simulink model "course project"  (R2023b)
settings: Solver=VariableStepAuto  StartTime=0.0  StopTime=2  RelTol=1e-3
libraries: simulink x1
(part 1 of 2)
settings Model: Creator=1234  LastModifiedBy=1234

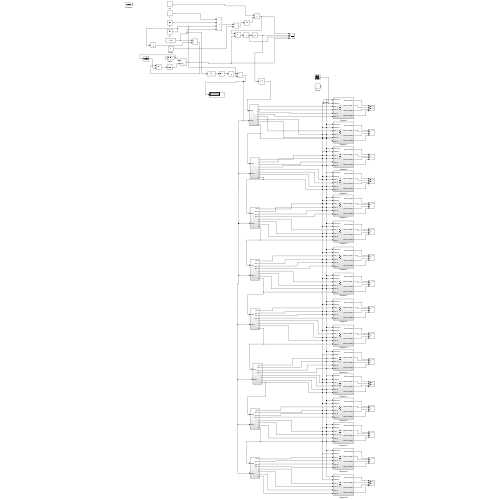
[thumbnail: Simulink's stored preview of the top-level diagram]
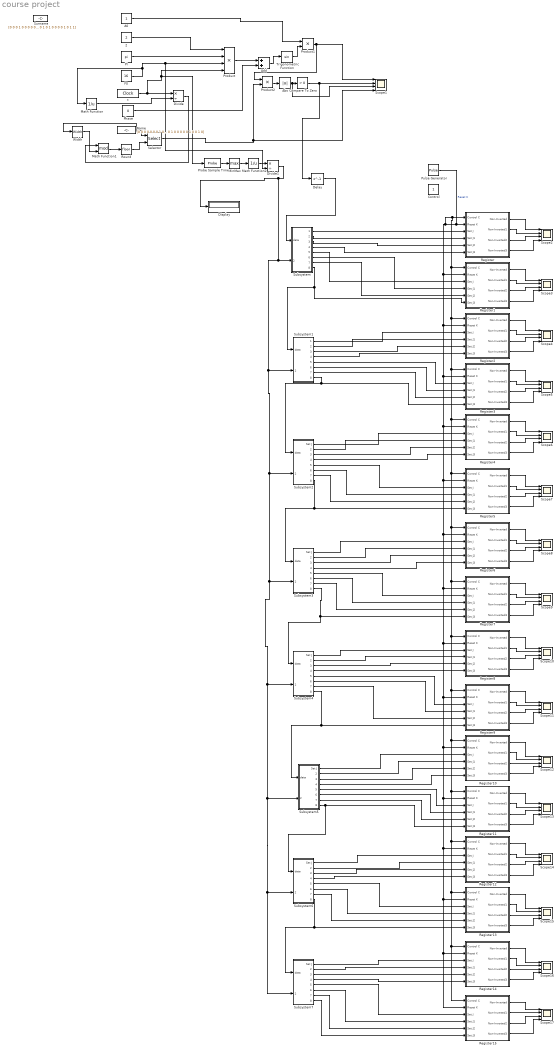
== system course project ==
  2 : Constant  Value=2
  A0 : Constant
  Abs : Abs  SaturateOnIntegerOverflow=off
  Add : Sum
  Compare To Zero : simulink/Logic and Bit Operations/Compare To Zero  relop=>  OutDataTypeStr=boolean
  Control : Constant
  Delay : Delay  DelayLength=1  InitialCondition=0
  Display : Display
  Divide : Product  Inputs=*/
  Divide1 : Product  Inputs=*/
  F0 : Constant  Value=16
  Math Function : Math  Operator=reciprocal
  Math Function1 : Math  Operator=mod
  Math Function2 : Math  Operator=reciprocal
  MinMax : MinMax  Function=max
  Name : Constant  Value=[0 0 0 0 0 0 0 1 0 0 0 0 1 1 0 0 0 0 0 0 0 1 0 1 0 0 0 1 1 0 0 0 0 0 0 0 0 0 0 1 0 0 0 0 1 1 1 0 0 0 0 0 0 1 0 0 0 0 0 1 0 0 1 0]  VectorParams1D=off
  PI : Constant  Value=pi
  Phase : Constant  Value=0
  Probe Sample Time : Probe  ProbeWidth=off  ProbeComplexSignal=off
  Product : Product  Inputs=4
  Product1 : Product
  Product2 : Product
  Pulse Generator : DiscretePulseGenerator  PulseType=Time based  PulseWidth=50
  Register : Subsystem
  Register1 : Subsystem
  Register10 : Subsystem
  Register11 : Subsystem
  Register12 : Subsystem
  Register13 : Subsystem
  Register14 : Subsystem
  Register15 : Subsystem
  Register2 : Subsystem
  Register3 : Subsystem
  Register4 : Subsystem
  Register5 : Subsystem
  Register6 : Subsystem
  Register7 : Subsystem
  Register8 : Subsystem
  Register9 : Subsystem
  Round : Rounding
  Scope{1..17} (17 alike) : Scope  NumInputPorts=4
  Selector : Selector  IndexMode=Zero-based  InputPortWidth=64  IndexOptions=Index vector (port)  Indices=[1 3]  OutputSizes=1
  Subsystem : Subsystem
  Subsystem1 : Subsystem
  Subsystem2 : Subsystem
  Subsystem3 : Subsystem
  Subsystem4 : Subsystem
  Subsystem5 : Subsystem
  Subsystem6 : Subsystem
  Subsystem7 : Subsystem
  Surname : Constant  Value=[0 0 0 1 0 0 0 0 0 0 0 0 1 1 1 1 0 0 0 0 0 1 1 1 0 0 0 1 0 0 1 0 0 0 0 0 0 1 0 1 0 0 0 0 0 0 1 0 0 0 0 0 1 1 1 0 0 0 0 1 1 0 0 1 0 0 0 1 0 1 0 1 0 0 0 0 1 0 1 1]
  Trigonometric Function : Trigonometry
  Width : Width
  t : DigitalClock  SampleTime=1/1000
  wires:
  Subsystem4/8(Out8) -> Register9/6(Set J3), Subsystem5/1(data)
  Trigonometric Function/1 -> Product1/2
  PI/1 -> Product/2
  A0/1 -> Product1/1
  MinMax/1 -> Math Function2/1
  Math Function1/1 -> Round/1
  Probe Sample Time/1 -> MinMax/1
  Product/1 -> Add/1
  Selector/1 -> Product2/2, Scope1/4
  Abs/1 -> Scope1/3, Compare To Zero/1
  Name/1 -> Width/1, Selector/1
  Subsystem1/8(Out8) -> Subsystem2/1(data), Register3/6(Set J3)
  Product2/1 -> Abs/1
  Product1/1 -> Scope1/1, Product2/1
  Phase/1 -> Add/2
  Subsystem6/8(Out8) -> Register13/6(Set J3), Subsystem7/1(data)
  Width/1 -> Math Function1/2
  Divide/1 -> Math Function1/1
  Math Function/1 -> Divide/2
  Compare To Zero/1 -> Delay/1, Scope1/2
  Round/1 -> Selector/2
  t/1 -> Probe Sample Time/1, Product/4, Divide/1
  2/1 -> Product/1
  Math Function2/1 -> Divide1/1
  F0/1 -> Math Function/1, Divide1/2, Product/3
  Subsystem/8(Out8) -> Register1/6(Set J3), Subsystem1/1(data)
  Delay/1 -> Subsystem/1(data)
  Subsystem5/8(Out8) -> Subsystem6/1(data), Register11/6(Set J3)
  Add/1 -> Trigonometric Function/1
  Subsystem2/8(Out8) -> Register5/6(Set J3), Subsystem3/1(data)
  Subsystem3/8(Out8) -> Register7/6(Set J3), Subsystem4/1(data)
  Subsystem/1(1) -> Register/3(Set J)
  Subsystem/2(2) -> Register/4(Set J1)
  Subsystem/3(3) -> Register/5(Set J2)
  Subsystem/4(4) -> Register/6(Set J3)
  Subsystem/5(Out5) -> Register1/3(Set J)
  Subsystem/6(Out6) -> Register1/4(Set J1)
  Subsystem/7(Out7) -> Register1/5(Set J2)
  Subsystem1/1(1) -> Register2/3(Set J)
  Subsystem1/2(2) -> Register2/4(Set J1)
  Subsystem1/3(3) -> Register2/5(Set J2)
  Subsystem1/4(4) -> Register2/6(Set J3)
  Subsystem1/5(Out5) -> Register3/3(Set J)
  Subsystem1/6(Out6) -> Register3/4(Set J1)
  Subsystem1/7(Out7) -> Register3/5(Set J2)
  Subsystem2/1(Set J) -> Register4/3(Set J)
  Subsystem2/2(Set J1) -> Register4/4(Set J1)
  Subsystem2/3(Set J2) -> Register4/5(Set J2)
  Subsystem2/4(Set J3) -> Register4/6(Set J3)
  Subsystem2/5(Out5) -> Register5/3(Set J)
  Subsystem2/6(Out6) -> Register5/4(Set J1)
  Subsystem2/7(Out7) -> Register5/5(Set J2)
  Subsystem3/1(Set J) -> Register6/3(Set J)
  Subsystem3/2(Set J1) -> Register6/4(Set J1)
  Subsystem3/3(Set J2) -> Register6/5(Set J2)
  Subsystem3/4(Set J3) -> Register6/6(Set J3)
  Subsystem3/5(Out5) -> Register7/3(Set J)
  Subsystem3/6(Out6) -> Register7/4(Set J1)
  Subsystem3/7(Out7) -> Register7/5(Set J2)
  Subsystem4/1(Set J) -> Register8/3(Set J)
  Subsystem4/2(Set J1) -> Register8/4(Set J1)
  Subsystem4/3(Set J2) -> Register8/5(Set J2)
  Subsystem4/4(Set J3) -> Register8/6(Set J3)
  Subsystem4/5(Out5) -> Register9/3(Set J)
  Subsystem4/6(Out6) -> Register9/4(Set J1)
  Subsystem4/7(Out7) -> Register9/5(Set J2)
  Subsystem5/1(Set J) -> Register10/3(Set J)
  Subsystem5/2(Set J1) -> Register10/4(Set J1)
  Subsystem5/3(Set J2) -> Register10/5(Set J2)
  Subsystem5/4(Set J3) -> Register10/6(Set J3)
  Subsystem5/5(Out5) -> Register11/3(Set J)
  Subsystem5/6(Out6) -> Register11/4(Set J1)
  Subsystem5/7(Out7) -> Register11/5(Set J2)
  Subsystem6/1(Set J) -> Register12/3(Set J)
  Subsystem6/2(Set J1) -> Register12/4(Set J1)
  Subsystem6/3(Set J2) -> Register12/5(Set J2)
  Subsystem6/4(Set J3) -> Register12/6(Set J3)
  Subsystem6/5(Out5) -> Register13/3(Set J)
  Subsystem6/6(Out6) -> Register13/4(Set J1)
  Subsystem6/7(Out7) -> Register13/5(Set J2)
  Subsystem7/1(Set J) -> Register14/3(Set J)
  Subsystem7/2(Set J1) -> Register14/4(Set J1)
  Subsystem7/3(Set J2) -> Register14/5(Set J2)
  Subsystem7/4(Set J3) -> Register14/6(Set J3)
  Subsystem7/5(Out5) -> Register15/3(Set J)
  Subsystem7/6(Out6) -> Register15/4(Set J1)
  Subsystem7/7(Out7) -> Register15/5(Set J2)
  Subsystem7/8(Out8) -> Register15/6(Set J3)
  Register/1(Non-Inverted) -> Scope2/1
  Register/2(Non-Inverted1) -> Scope2/2
  Register/3(Non-Inverted2) -> Scope2/3
  Register/4(Non-Inverted3) -> Scope2/4
  Register1/3(Non-Inverted2) -> Scope3/3
  Register1/4(Non-Inverted3) -> Scope3/4
  Register1/2(Non-Inverted1) -> Scope3/2
  Register1/1(Non-Inverted) -> Scope3/1
  Register2/3(Non-Inverted2) -> Scope4/3
  Register2/4(Non-Inverted3) -> Scope4/4
  Register2/2(Non-Inverted1) -> Scope4/2
  Register2/1(Non-Inverted) -> Scope4/1
  Register3/3(Non-Inverted2) -> Scope5/3
  Register3/4(Non-Inverted3) -> Scope5/4
  Register3/2(Non-Inverted1) -> Scope5/2
  Register3/1(Non-Inverted) -> Scope5/1
  Register4/3(Non-Inverted2) -> Scope6/3
  Register4/4(Non-Inverted3) -> Scope6/4
  Register4/2(Non-Inverted1) -> Scope6/2
  Register4/1(Non-Inverted) -> Scope6/1
  Register5/3(Non-Inverted2) -> Scope7/3
  Register5/4(Non-Inverted3) -> Scope7/4
  Register5/2(Non-Inverted1) -> Scope7/2
  Register5/1(Non-Inverted) -> Scope7/1
  Register6/3(Non-Inverted2) -> Scope8/3
  Register6/4(Non-Inverted3) -> Scope8/4
  Register6/2(Non-Inverted1) -> Scope8/2
  Register6/1(Non-Inverted) -> Scope8/1
  Register7/3(Non-Inverted2) -> Scope9/3
  Register7/4(Non-Inverted3) -> Scope9/4
  Register7/2(Non-Inverted1) -> Scope9/2
  Register7/1(Non-Inverted) -> Scope9/1
  Register8/3(Non-Inverted2) -> Scope10/3
  Register8/4(Non-Inverted3) -> Scope10/4
  Register8/2(Non-Inverted1) -> Scope10/2
  Register8/1(Non-Inverted) -> Scope10/1
  Register9/3(Non-Inverted2) -> Scope11/3
  Register9/4(Non-Inverted3) -> Scope11/4
  Register9/2(Non-Inverted1) -> Scope11/2
  Register9/1(Non-Inverted) -> Scope11/1
  Register10/1(Non-Inverted) -> Scope12/1
  Register10/2(Non-Inverted1) -> Scope12/2
  Register10/3(Non-Inverted2) -> Scope12/3
  Register10/4(Non-Inverted3) -> Scope12/4
  Register11/1(Non-Inverted) -> Scope13/1
  Register11/2(Non-Inverted1) -> Scope13/2
  Register11/3(Non-Inverted2) -> Scope13/3
  Register11/4(Non-Inverted3) -> Scope13/4
  Register15/1(Non-Inverted) -> Scope17/1
  Register15/2(Non-Inverted1) -> Scope17/2
  Register15/4(Non-Inverted3) -> Scope17/4
  Register14/4(Non-Inverted3) -> Scope16/4
  Register14/1(Non-Inverted) -> Scope16/1
  Register14/2(Non-Inverted1) -> Scope16/2
  Register14/3(Non-Inverted2) -> Scope16/3
  Register15/3(Non-Inverted2) -> Scope17/3
  Register12/2(Non-Inverted1) -> Scope14/2
  Register12/1(Non-Inverted) -> Scope14/1
  Register13/1(Non-Inverted) -> Scope15/1
  Register13/2(Non-Inverted1) -> Scope15/2
  Register12/4(Non-Inverted3) -> Scope14/4
  Register13/3(Non-Inverted2) -> Scope15/3
  Register12/3(Non-Inverted2) -> Scope14/3
  Register13/4(Non-Inverted3) -> Scope15/4
  Divide1/1 -> Display/1, Subsystem7/2(delay), Subsystem6/2(delay), Subsystem5/2(delay), Subsystem4/2(delay), Subsystem3/2(delay), Subsystem2/2(delay), Subsystem1/2(delay), Subsystem/2(delay)
  Pulse Generator/1 -> Register1/1(Control C), Register2/1(Control C), Register3/1(Control C), Register4/1(Control C), Register5/1(Control C), Register6/1(Control C), Register7/1(Control C), Register8/1(Control C), Register9/1(Control C), Register10/1(Control C), Register11/1(Control C), Register12/1(Control C), Register13/1(Control C), Register14/1(Control C), Register15/1(Control C), Register/1(Control C), Register15/2(Reset K), Register14/2(Reset K), Register13/2(Reset K), Register12/2(Reset K), Register11/2(Reset K), Register10/2(Reset K), Register9/2(Reset K), Register8/2(Reset K), Register7/2(Reset K), Register6/2(Reset K), Register5/2(Reset K), Register4/2(Reset K), Register3/2(Reset K), Register2/2(Reset K), Register1/2(Reset K), Register/2(Reset K)  "Reset K"

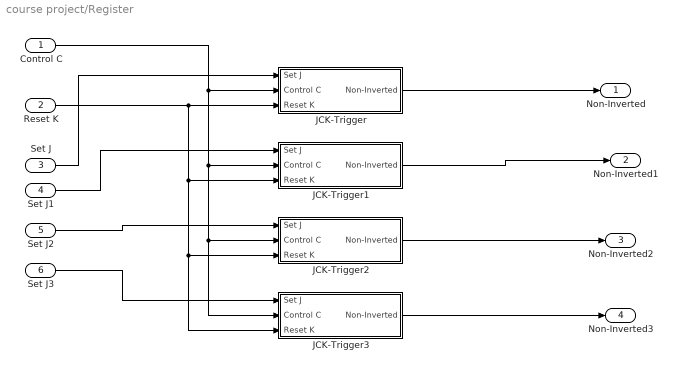
== system course project/Register ==
  Control C : Inport
  Reset K : Inport  Port=2
  Set J : Inport  Port=3
  Set J1 : Inport  Port=4
  Set J2 : Inport  Port=5
  Set J3 : Inport  Port=6
  JCK-Trigger : Subsystem
  JCK-Trigger1 : Subsystem
  JCK-Trigger2 : Subsystem
  JCK-Trigger3 : Subsystem
  Non-Inverted : Outport
  Non-Inverted1 : Outport  Port=2
  Non-Inverted2 : Outport  Port=3
  Non-Inverted3 : Outport  Port=4
  wires:
  JCK-Trigger3/1(Non-Inverted) -> Non-Inverted3/1
  Control C/1 -> JCK-Trigger3/2(Control C), JCK-Trigger2/2(Control C), JCK-Trigger1/2(Control C), JCK-Trigger/2(Control C)
  Reset K/1 -> JCK-Trigger3/3(Reset K), JCK-Trigger2/3(Reset K), JCK-Trigger1/3(Reset K), JCK-Trigger/3(Reset K)
  Set J3/1 -> JCK-Trigger3/1(Set J)
  JCK-Trigger2/1(Non-Inverted) -> Non-Inverted2/1
  Set J1/1 -> JCK-Trigger1/1(Set J)
  Set J2/1 -> JCK-Trigger2/1(Set J)
  Set J/1 -> JCK-Trigger/1(Set J)
  JCK-Trigger1/1(Non-Inverted) -> Non-Inverted1/1
  JCK-Trigger/1(Non-Inverted) -> Non-Inverted/1

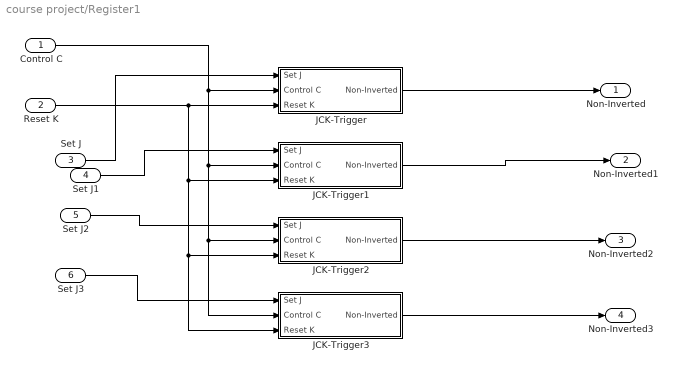
== system course project/Register1 ==
  Control C : Inport
  Reset K : Inport  Port=2
  Set J : Inport  Port=3
  Set J1 : Inport  Port=4
  Set J2 : Inport  Port=5
  Set J3 : Inport  Port=6
  JCK-Trigger : Subsystem
  JCK-Trigger1 : Subsystem
  JCK-Trigger2 : Subsystem
  JCK-Trigger3 : Subsystem
  Non-Inverted : Outport
  Non-Inverted1 : Outport  Port=2
  Non-Inverted2 : Outport  Port=3
  Non-Inverted3 : Outport  Port=4
  wires:
  JCK-Trigger3/1(Non-Inverted) -> Non-Inverted3/1
  Control C/1 -> JCK-Trigger3/2(Control C), JCK-Trigger2/2(Control C), JCK-Trigger1/2(Control C), JCK-Trigger/2(Control C)
  Reset K/1 -> JCK-Trigger3/3(Reset K), JCK-Trigger2/3(Reset K), JCK-Trigger1/3(Reset K), JCK-Trigger/3(Reset K)
  Set J3/1 -> JCK-Trigger3/1(Set J)
  JCK-Trigger2/1(Non-Inverted) -> Non-Inverted2/1
  Set J1/1 -> JCK-Trigger1/1(Set J)
  Set J2/1 -> JCK-Trigger2/1(Set J)
  Set J/1 -> JCK-Trigger/1(Set J)
  JCK-Trigger1/1(Non-Inverted) -> Non-Inverted1/1
  JCK-Trigger/1(Non-Inverted) -> Non-Inverted/1

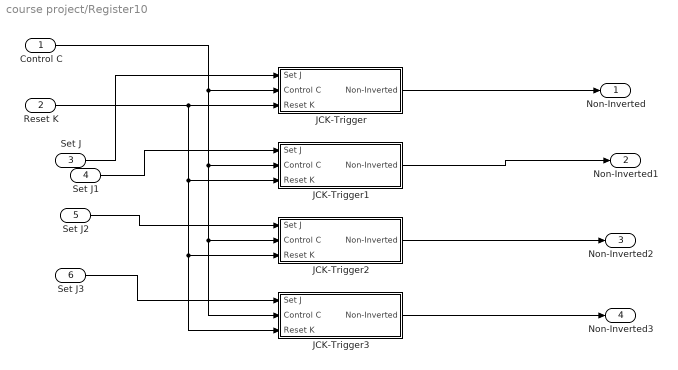
== system course project/Register10 ==
  Control C : Inport
  Reset K : Inport  Port=2
  Set J : Inport  Port=3
  Set J1 : Inport  Port=4
  Set J2 : Inport  Port=5
  Set J3 : Inport  Port=6
  JCK-Trigger : Subsystem
  JCK-Trigger1 : Subsystem
  JCK-Trigger2 : Subsystem
  JCK-Trigger3 : Subsystem
  Non-Inverted : Outport
  Non-Inverted1 : Outport  Port=2
  Non-Inverted2 : Outport  Port=3
  Non-Inverted3 : Outport  Port=4
  wires:
  JCK-Trigger3/1(Non-Inverted) -> Non-Inverted3/1
  Control C/1 -> JCK-Trigger3/2(Control C), JCK-Trigger2/2(Control C), JCK-Trigger1/2(Control C), JCK-Trigger/2(Control C)
  Reset K/1 -> JCK-Trigger3/3(Reset K), JCK-Trigger2/3(Reset K), JCK-Trigger1/3(Reset K), JCK-Trigger/3(Reset K)
  Set J3/1 -> JCK-Trigger3/1(Set J)
  JCK-Trigger2/1(Non-Inverted) -> Non-Inverted2/1
  Set J1/1 -> JCK-Trigger1/1(Set J)
  Set J2/1 -> JCK-Trigger2/1(Set J)
  Set J/1 -> JCK-Trigger/1(Set J)
  JCK-Trigger1/1(Non-Inverted) -> Non-Inverted1/1
  JCK-Trigger/1(Non-Inverted) -> Non-Inverted/1

== system course project/Register11 ==
  Control C : Inport
  Reset K : Inport  Port=2
  Set J : Inport  Port=3
  Set J1 : Inport  Port=4
  Set J2 : Inport  Port=5
  Set J3 : Inport  Port=6
  JCK-Trigger : Subsystem
  JCK-Trigger1 : Subsystem
  JCK-Trigger2 : Subsystem
  JCK-Trigger3 : Subsystem
  Non-Inverted : Outport
  Non-Inverted1 : Outport  Port=2
  Non-Inverted2 : Outport  Port=3
  Non-Inverted3 : Outport  Port=4
  wires:
  JCK-Trigger3/1(Non-Inverted) -> Non-Inverted3/1
  Control C/1 -> JCK-Trigger3/2(Control C), JCK-Trigger2/2(Control C), JCK-Trigger1/2(Control C), JCK-Trigger/2(Control C)
  Reset K/1 -> JCK-Trigger3/3(Reset K), JCK-Trigger2/3(Reset K), JCK-Trigger1/3(Reset K), JCK-Trigger/3(Reset K)
  Set J3/1 -> JCK-Trigger3/1(Set J)
  JCK-Trigger2/1(Non-Inverted) -> Non-Inverted2/1
  Set J1/1 -> JCK-Trigger1/1(Set J)
  Set J2/1 -> JCK-Trigger2/1(Set J)
  Set J/1 -> JCK-Trigger/1(Set J)
  JCK-Trigger1/1(Non-Inverted) -> Non-Inverted1/1
  JCK-Trigger/1(Non-Inverted) -> Non-Inverted/1

== system course project/Register12 ==
  Control C : Inport
  Reset K : Inport  Port=2
  Set J : Inport  Port=3
  Set J1 : Inport  Port=4
  Set J2 : Inport  Port=5
  Set J3 : Inport  Port=6
  JCK-Trigger : Subsystem
  JCK-Trigger1 : Subsystem
  JCK-Trigger2 : Subsystem
  JCK-Trigger3 : Subsystem
  Non-Inverted : Outport
  Non-Inverted1 : Outport  Port=2
  Non-Inverted2 : Outport  Port=3
  Non-Inverted3 : Outport  Port=4
  wires:
  JCK-Trigger3/1(Non-Inverted) -> Non-Inverted3/1
  Control C/1 -> JCK-Trigger3/2(Control C), JCK-Trigger2/2(Control C), JCK-Trigger1/2(Control C), JCK-Trigger/2(Control C)
  Reset K/1 -> JCK-Trigger3/3(Reset K), JCK-Trigger2/3(Reset K), JCK-Trigger1/3(Reset K), JCK-Trigger/3(Reset K)
  Set J3/1 -> JCK-Trigger3/1(Set J)
  JCK-Trigger2/1(Non-Inverted) -> Non-Inverted2/1
  Set J1/1 -> JCK-Trigger1/1(Set J)
  Set J2/1 -> JCK-Trigger2/1(Set J)
  Set J/1 -> JCK-Trigger/1(Set J)
  JCK-Trigger1/1(Non-Inverted) -> Non-Inverted1/1
  JCK-Trigger/1(Non-Inverted) -> Non-Inverted/1

== system course project/Register13 ==
  Control C : Inport
  Reset K : Inport  Port=2
  Set J : Inport  Port=3
  Set J1 : Inport  Port=4
  Set J2 : Inport  Port=5
  Set J3 : Inport  Port=6
  JCK-Trigger : Subsystem
  JCK-Trigger1 : Subsystem
  JCK-Trigger2 : Subsystem
  JCK-Trigger3 : Subsystem
  Non-Inverted : Outport
  Non-Inverted1 : Outport  Port=2
  Non-Inverted2 : Outport  Port=3
  Non-Inverted3 : Outport  Port=4
  wires:
  JCK-Trigger3/1(Non-Inverted) -> Non-Inverted3/1
  Control C/1 -> JCK-Trigger3/2(Control C), JCK-Trigger2/2(Control C), JCK-Trigger1/2(Control C), JCK-Trigger/2(Control C)
  Reset K/1 -> JCK-Trigger3/3(Reset K), JCK-Trigger2/3(Reset K), JCK-Trigger1/3(Reset K), JCK-Trigger/3(Reset K)
  Set J3/1 -> JCK-Trigger3/1(Set J)
  JCK-Trigger2/1(Non-Inverted) -> Non-Inverted2/1
  Set J1/1 -> JCK-Trigger1/1(Set J)
  Set J2/1 -> JCK-Trigger2/1(Set J)
  Set J/1 -> JCK-Trigger/1(Set J)
  JCK-Trigger1/1(Non-Inverted) -> Non-Inverted1/1
  JCK-Trigger/1(Non-Inverted) -> Non-Inverted/1

== system course project/Register14 ==
  Control C : Inport
  Reset K : Inport  Port=2
  Set J : Inport  Port=3
  Set J1 : Inport  Port=4
  Set J2 : Inport  Port=5
  Set J3 : Inport  Port=6
  JCK-Trigger : Subsystem
  JCK-Trigger1 : Subsystem
  JCK-Trigger2 : Subsystem
  JCK-Trigger3 : Subsystem
  Non-Inverted : Outport
  Non-Inverted1 : Outport  Port=2
  Non-Inverted2 : Outport  Port=3
  Non-Inverted3 : Outport  Port=4
  wires:
  JCK-Trigger3/1(Non-Inverted) -> Non-Inverted3/1
  Control C/1 -> JCK-Trigger3/2(Control C), JCK-Trigger2/2(Control C), JCK-Trigger1/2(Control C), JCK-Trigger/2(Control C)
  Reset K/1 -> JCK-Trigger3/3(Reset K), JCK-Trigger2/3(Reset K), JCK-Trigger1/3(Reset K), JCK-Trigger/3(Reset K)
  Set J3/1 -> JCK-Trigger3/1(Set J)
  JCK-Trigger2/1(Non-Inverted) -> Non-Inverted2/1
  Set J1/1 -> JCK-Trigger1/1(Set J)
  Set J2/1 -> JCK-Trigger2/1(Set J)
  Set J/1 -> JCK-Trigger/1(Set J)
  JCK-Trigger1/1(Non-Inverted) -> Non-Inverted1/1
  JCK-Trigger/1(Non-Inverted) -> Non-Inverted/1

== system course project/Register15 ==
  Control C : Inport
  Reset K : Inport  Port=2
  Set J : Inport  Port=3
  Set J1 : Inport  Port=4
  Set J2 : Inport  Port=5
  Set J3 : Inport  Port=6
  JCK-Trigger : Subsystem
  JCK-Trigger1 : Subsystem
  JCK-Trigger2 : Subsystem
  JCK-Trigger3 : Subsystem
  Non-Inverted : Outport
  Non-Inverted1 : Outport  Port=2
  Non-Inverted2 : Outport  Port=3
  Non-Inverted3 : Outport  Port=4
  wires:
  JCK-Trigger3/1(Non-Inverted) -> Non-Inverted3/1
  Control C/1 -> JCK-Trigger3/2(Control C), JCK-Trigger2/2(Control C), JCK-Trigger1/2(Control C), JCK-Trigger/2(Control C)
  Reset K/1 -> JCK-Trigger3/3(Reset K), JCK-Trigger2/3(Reset K), JCK-Trigger1/3(Reset K), JCK-Trigger/3(Reset K)
  Set J3/1 -> JCK-Trigger3/1(Set J)
  JCK-Trigger2/1(Non-Inverted) -> Non-Inverted2/1
  Set J1/1 -> JCK-Trigger1/1(Set J)
  Set J2/1 -> JCK-Trigger2/1(Set J)
  Set J/1 -> JCK-Trigger/1(Set J)
  JCK-Trigger1/1(Non-Inverted) -> Non-Inverted1/1
  JCK-Trigger/1(Non-Inverted) -> Non-Inverted/1

== system course project/Register2 ==
  Control C : Inport
  Reset K : Inport  Port=2
  Set J : Inport  Port=3
  Set J1 : Inport  Port=4
  Set J2 : Inport  Port=5
  Set J3 : Inport  Port=6
  JCK-Trigger : Subsystem
  JCK-Trigger1 : Subsystem
  JCK-Trigger2 : Subsystem
  JCK-Trigger3 : Subsystem
  Non-Inverted : Outport
  Non-Inverted1 : Outport  Port=2
  Non-Inverted2 : Outport  Port=3
  Non-Inverted3 : Outport  Port=4
  wires:
  JCK-Trigger3/1(Non-Inverted) -> Non-Inverted3/1
  Control C/1 -> JCK-Trigger3/2(Control C), JCK-Trigger2/2(Control C), JCK-Trigger1/2(Control C), JCK-Trigger/2(Control C)
  Reset K/1 -> JCK-Trigger3/3(Reset K), JCK-Trigger2/3(Reset K), JCK-Trigger1/3(Reset K), JCK-Trigger/3(Reset K)
  Set J3/1 -> JCK-Trigger3/1(Set J)
  JCK-Trigger2/1(Non-Inverted) -> Non-Inverted2/1
  Set J1/1 -> JCK-Trigger1/1(Set J)
  Set J2/1 -> JCK-Trigger2/1(Set J)
  Set J/1 -> JCK-Trigger/1(Set J)
  JCK-Trigger1/1(Non-Inverted) -> Non-Inverted1/1
  JCK-Trigger/1(Non-Inverted) -> Non-Inverted/1

== system course project/Register3 ==
  Control C : Inport
  Reset K : Inport  Port=2
  Set J : Inport  Port=3
  Set J1 : Inport  Port=4
  Set J2 : Inport  Port=5
  Set J3 : Inport  Port=6
  JCK-Trigger : Subsystem
  JCK-Trigger1 : Subsystem
  JCK-Trigger2 : Subsystem
  JCK-Trigger3 : Subsystem
  Non-Inverted : Outport
  Non-Inverted1 : Outport  Port=2
  Non-Inverted2 : Outport  Port=3
  Non-Inverted3 : Outport  Port=4
  wires:
  JCK-Trigger3/1(Non-Inverted) -> Non-Inverted3/1
  Control C/1 -> JCK-Trigger3/2(Control C), JCK-Trigger2/2(Control C), JCK-Trigger1/2(Control C), JCK-Trigger/2(Control C)
  Reset K/1 -> JCK-Trigger3/3(Reset K), JCK-Trigger2/3(Reset K), JCK-Trigger1/3(Reset K), JCK-Trigger/3(Reset K)
  Set J3/1 -> JCK-Trigger3/1(Set J)
  JCK-Trigger2/1(Non-Inverted) -> Non-Inverted2/1
  Set J1/1 -> JCK-Trigger1/1(Set J)
  Set J2/1 -> JCK-Trigger2/1(Set J)
  Set J/1 -> JCK-Trigger/1(Set J)
  JCK-Trigger1/1(Non-Inverted) -> Non-Inverted1/1
  JCK-Trigger/1(Non-Inverted) -> Non-Inverted/1

== system course project/Register4 ==
  Control C : Inport
  Reset K : Inport  Port=2
  Set J : Inport  Port=3
  Set J1 : Inport  Port=4
  Set J2 : Inport  Port=5
  Set J3 : Inport  Port=6
  JCK-Trigger : Subsystem
  JCK-Trigger1 : Subsystem
  JCK-Trigger2 : Subsystem
  JCK-Trigger3 : Subsystem
  Non-Inverted : Outport
  Non-Inverted1 : Outport  Port=2
  Non-Inverted2 : Outport  Port=3
  Non-Inverted3 : Outport  Port=4
  wires:
  JCK-Trigger3/1(Non-Inverted) -> Non-Inverted3/1
  Control C/1 -> JCK-Trigger3/2(Control C), JCK-Trigger2/2(Control C), JCK-Trigger1/2(Control C), JCK-Trigger/2(Control C)
  Reset K/1 -> JCK-Trigger3/3(Reset K), JCK-Trigger2/3(Reset K), JCK-Trigger1/3(Reset K), JCK-Trigger/3(Reset K)
  Set J3/1 -> JCK-Trigger3/1(Set J)
  JCK-Trigger2/1(Non-Inverted) -> Non-Inverted2/1
  Set J1/1 -> JCK-Trigger1/1(Set J)
  Set J2/1 -> JCK-Trigger2/1(Set J)
  Set J/1 -> JCK-Trigger/1(Set J)
  JCK-Trigger1/1(Non-Inverted) -> Non-Inverted1/1
  JCK-Trigger/1(Non-Inverted) -> Non-Inverted/1

== system course project/Register5 ==
  Control C : Inport
  Reset K : Inport  Port=2
  Set J : Inport  Port=3
  Set J1 : Inport  Port=4
  Set J2 : Inport  Port=5
  Set J3 : Inport  Port=6
  JCK-Trigger : Subsystem
  JCK-Trigger1 : Subsystem
  JCK-Trigger2 : Subsystem
  JCK-Trigger3 : Subsystem
  Non-Inverted : Outport
  Non-Inverted1 : Outport  Port=2
  Non-Inverted2 : Outport  Port=3
  Non-Inverted3 : Outport  Port=4
  wires:
  JCK-Trigger3/1(Non-Inverted) -> Non-Inverted3/1
  Control C/1 -> JCK-Trigger3/2(Control C), JCK-Trigger2/2(Control C), JCK-Trigger1/2(Control C), JCK-Trigger/2(Control C)
  Reset K/1 -> JCK-Trigger3/3(Reset K), JCK-Trigger2/3(Reset K), JCK-Trigger1/3(Reset K), JCK-Trigger/3(Reset K)
  Set J3/1 -> JCK-Trigger3/1(Set J)
  JCK-Trigger2/1(Non-Inverted) -> Non-Inverted2/1
  Set J1/1 -> JCK-Trigger1/1(Set J)
  Set J2/1 -> JCK-Trigger2/1(Set J)
  Set J/1 -> JCK-Trigger/1(Set J)
  JCK-Trigger1/1(Non-Inverted) -> Non-Inverted1/1
  JCK-Trigger/1(Non-Inverted) -> Non-Inverted/1

== system course project/Register6 ==
  Control C : Inport
  Reset K : Inport  Port=2
  Set J : Inport  Port=3
  Set J1 : Inport  Port=4
  Set J2 : Inport  Port=5
  Set J3 : Inport  Port=6
  JCK-Trigger : Subsystem
  JCK-Trigger1 : Subsystem
  JCK-Trigger2 : Subsystem
  JCK-Trigger3 : Subsystem
  Non-Inverted : Outport
  Non-Inverted1 : Outport  Port=2
  Non-Inverted2 : Outport  Port=3
  Non-Inverted3 : Outport  Port=4
  wires:
  JCK-Trigger3/1(Non-Inverted) -> Non-Inverted3/1
  Control C/1 -> JCK-Trigger3/2(Control C), JCK-Trigger2/2(Control C), JCK-Trigger1/2(Control C), JCK-Trigger/2(Control C)
  Reset K/1 -> JCK-Trigger3/3(Reset K), JCK-Trigger2/3(Reset K), JCK-Trigger1/3(Reset K), JCK-Trigger/3(Reset K)
  Set J3/1 -> JCK-Trigger3/1(Set J)
  JCK-Trigger2/1(Non-Inverted) -> Non-Inverted2/1
  Set J1/1 -> JCK-Trigger1/1(Set J)
  Set J2/1 -> JCK-Trigger2/1(Set J)
  Set J/1 -> JCK-Trigger/1(Set J)
  JCK-Trigger1/1(Non-Inverted) -> Non-Inverted1/1
  JCK-Trigger/1(Non-Inverted) -> Non-Inverted/1

== system course project/Register7 ==
  Control C : Inport
  Reset K : Inport  Port=2
  Set J : Inport  Port=3
  Set J1 : Inport  Port=4
  Set J2 : Inport  Port=5
  Set J3 : Inport  Port=6
  JCK-Trigger : Subsystem
  JCK-Trigger1 : Subsystem
  JCK-Trigger2 : Subsystem
  JCK-Trigger3 : Subsystem
  Non-Inverted : Outport
  Non-Inverted1 : Outport  Port=2
  Non-Inverted2 : Outport  Port=3
  Non-Inverted3 : Outport  Port=4
  wires:
  JCK-Trigger3/1(Non-Inverted) -> Non-Inverted3/1
  Control C/1 -> JCK-Trigger3/2(Control C), JCK-Trigger2/2(Control C), JCK-Trigger1/2(Control C), JCK-Trigger/2(Control C)
  Reset K/1 -> JCK-Trigger3/3(Reset K), JCK-Trigger2/3(Reset K), JCK-Trigger1/3(Reset K), JCK-Trigger/3(Reset K)
  Set J3/1 -> JCK-Trigger3/1(Set J)
  JCK-Trigger2/1(Non-Inverted) -> Non-Inverted2/1
  Set J1/1 -> JCK-Trigger1/1(Set J)
  Set J2/1 -> JCK-Trigger2/1(Set J)
  Set J/1 -> JCK-Trigger/1(Set J)
  JCK-Trigger1/1(Non-Inverted) -> Non-Inverted1/1
  JCK-Trigger/1(Non-Inverted) -> Non-Inverted/1

== system course project/Register8 ==
  Control C : Inport
  Reset K : Inport  Port=2
  Set J : Inport  Port=3
  Set J1 : Inport  Port=4
  Set J2 : Inport  Port=5
  Set J3 : Inport  Port=6
  JCK-Trigger : Subsystem
  JCK-Trigger1 : Subsystem
  JCK-Trigger2 : Subsystem
  JCK-Trigger3 : Subsystem
  Non-Inverted : Outport
  Non-Inverted1 : Outport  Port=2
  Non-Inverted2 : Outport  Port=3
  Non-Inverted3 : Outport  Port=4
  wires:
  JCK-Trigger3/1(Non-Inverted) -> Non-Inverted3/1
  Control C/1 -> JCK-Trigger3/2(Control C), JCK-Trigger2/2(Control C), JCK-Trigger1/2(Control C), JCK-Trigger/2(Control C)
  Reset K/1 -> JCK-Trigger3/3(Reset K), JCK-Trigger2/3(Reset K), JCK-Trigger1/3(Reset K), JCK-Trigger/3(Reset K)
  Set J3/1 -> JCK-Trigger3/1(Set J)
  JCK-Trigger2/1(Non-Inverted) -> Non-Inverted2/1
  Set J1/1 -> JCK-Trigger1/1(Set J)
  Set J2/1 -> JCK-Trigger2/1(Set J)
  Set J/1 -> JCK-Trigger/1(Set J)
  JCK-Trigger1/1(Non-Inverted) -> Non-Inverted1/1
  JCK-Trigger/1(Non-Inverted) -> Non-Inverted/1

== system course project/Register9 ==
  Control C : Inport
  Reset K : Inport  Port=2
  Set J : Inport  Port=3
  Set J1 : Inport  Port=4
  Set J2 : Inport  Port=5
  Set J3 : Inport  Port=6
  JCK-Trigger : Subsystem
  JCK-Trigger1 : Subsystem
  JCK-Trigger2 : Subsystem
  JCK-Trigger3 : Subsystem
  Non-Inverted : Outport
  Non-Inverted1 : Outport  Port=2
  Non-Inverted2 : Outport  Port=3
  Non-Inverted3 : Outport  Port=4
  wires:
  JCK-Trigger3/1(Non-Inverted) -> Non-Inverted3/1
  Control C/1 -> JCK-Trigger3/2(Control C), JCK-Trigger2/2(Control C), JCK-Trigger1/2(Control C), JCK-Trigger/2(Control C)
  Reset K/1 -> JCK-Trigger3/3(Reset K), JCK-Trigger2/3(Reset K), JCK-Trigger1/3(Reset K), JCK-Trigger/3(Reset K)
  Set J3/1 -> JCK-Trigger3/1(Set J)
  JCK-Trigger2/1(Non-Inverted) -> Non-Inverted2/1
  Set J1/1 -> JCK-Trigger1/1(Set J)
  Set J2/1 -> JCK-Trigger2/1(Set J)
  Set J/1 -> JCK-Trigger/1(Set J)
  JCK-Trigger1/1(Non-Inverted) -> Non-Inverted1/1
  JCK-Trigger/1(Non-Inverted) -> Non-Inverted/1

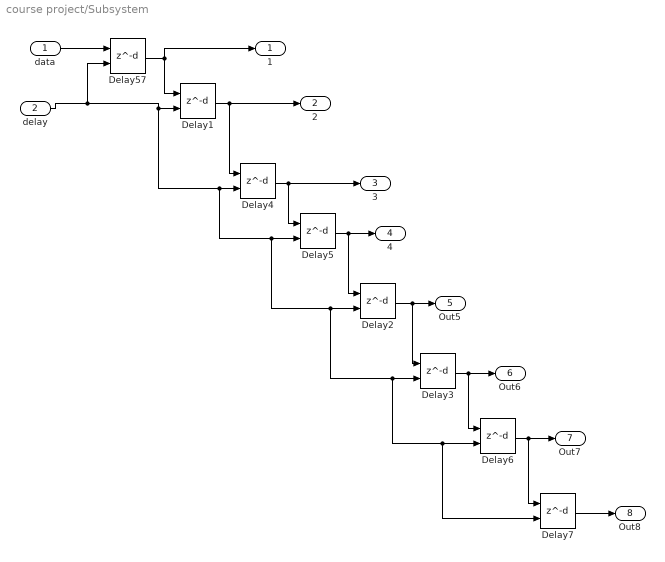
== system course project/Subsystem ==
  data : Inport
  delay : Inport  Port=2
  Delay{1..7,57} (8 alike) : Delay  DelayLengthSource=Input port  DelayLength=1  DelayLengthUpperLimit=2000  InitialCondition=0
      settings: InputPortMap=u0,p1
  1 : Outport
  2 : Outport  Port=2
  3 : Outport  Port=3
  4 : Outport  Port=4
  Out5 : Outport  Port=5
  Out6 : Outport  Port=6
  Out7 : Outport  Port=7
  Out8 : Outport  Port=8
  wires:
  Delay57/1 -> 1/1, Delay1/1
  Delay1/1 -> Delay4/1, 2/1
  Delay4/1 -> Delay5/1, 3/1
  Delay5/1 -> Delay2/1, 4/1
  Delay2/1 -> Delay3/1, Out5/1
  Delay3/1 -> Delay6/1, Out6/1
  Delay6/1 -> Delay7/1, Out7/1
  Delay7/1 -> Out8/1
  data/1 -> Delay57/1
  delay/1 -> Delay7/2, Delay6/2, Delay3/2, Delay2/2, Delay5/2, Delay4/2, Delay1/2, Delay57/2

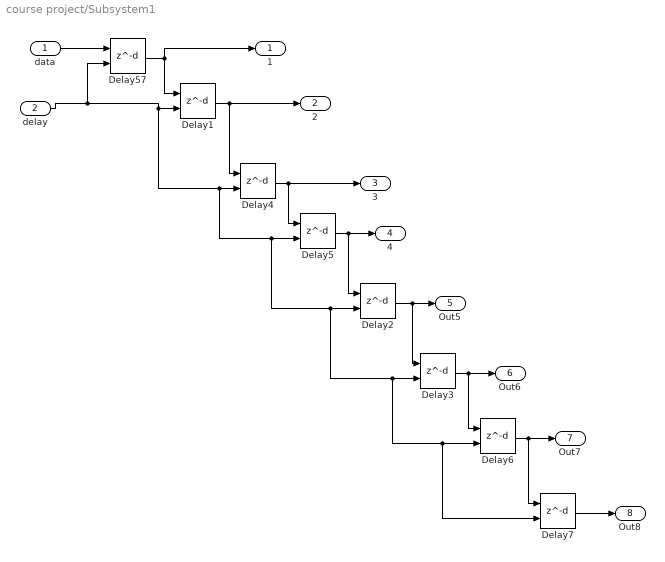
== system course project/Subsystem1 ==
  data : Inport
  delay : Inport  Port=2
  Delay{1..7,57} (8 alike) : Delay  DelayLengthSource=Input port  DelayLength=1  DelayLengthUpperLimit=2000  InitialCondition=0
      settings: InputPortMap=u0,p1
  1 : Outport
  2 : Outport  Port=2
  3 : Outport  Port=3
  4 : Outport  Port=4
  Out5 : Outport  Port=5
  Out6 : Outport  Port=6
  Out7 : Outport  Port=7
  Out8 : Outport  Port=8
  wires:
  Delay57/1 -> 1/1, Delay1/1
  Delay1/1 -> Delay4/1, 2/1
  Delay4/1 -> Delay5/1, 3/1
  Delay5/1 -> Delay2/1, 4/1
  Delay2/1 -> Delay3/1, Out5/1
  Delay3/1 -> Delay6/1, Out6/1
  Delay6/1 -> Delay7/1, Out7/1
  Delay7/1 -> Out8/1
  data/1 -> Delay57/1
  delay/1 -> Delay7/2, Delay6/2, Delay3/2, Delay2/2, Delay5/2, Delay4/2, Delay1/2, Delay57/2

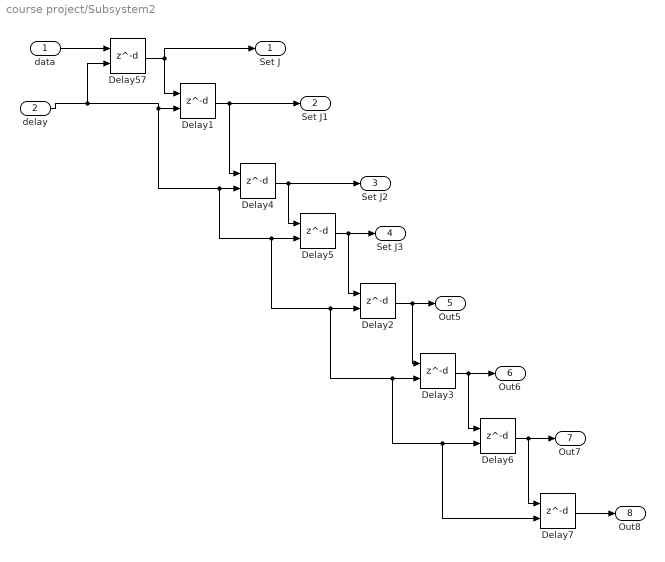
== system course project/Subsystem2 ==
  data : Inport
  delay : Inport  Port=2
  Delay{1..7,57} (8 alike) : Delay  DelayLengthSource=Input port  DelayLength=1  DelayLengthUpperLimit=2000  InitialCondition=0
      settings: InputPortMap=u0,p1
  Set J : Outport
  Set J1 : Outport  Port=2
  Set J2 : Outport  Port=3
  Set J3 : Outport  Port=4
  Out5 : Outport  Port=5
  Out6 : Outport  Port=6
  Out7 : Outport  Port=7
  Out8 : Outport  Port=8
  wires:
  Delay57/1 -> Set J/1, Delay1/1
  Delay1/1 -> Delay4/1, Set J1/1
  Delay4/1 -> Delay5/1, Set J2/1
  Delay5/1 -> Delay2/1, Set J3/1
  Delay2/1 -> Delay3/1, Out5/1
  Delay3/1 -> Delay6/1, Out6/1
  Delay6/1 -> Delay7/1, Out7/1
  Delay7/1 -> Out8/1
  data/1 -> Delay57/1
  delay/1 -> Delay7/2, Delay6/2, Delay3/2, Delay2/2, Delay5/2, Delay4/2, Delay1/2, Delay57/2

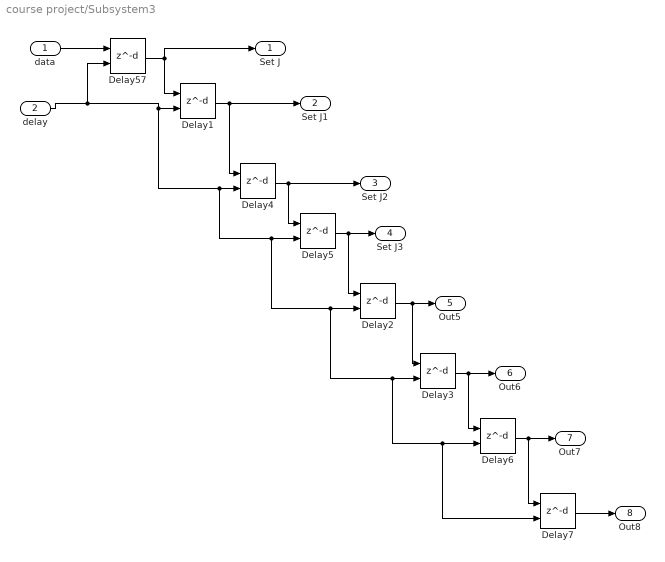
== system course project/Subsystem3 ==
  data : Inport
  delay : Inport  Port=2
  Delay{1..7,57} (8 alike) : Delay  DelayLengthSource=Input port  DelayLength=1  DelayLengthUpperLimit=2000  InitialCondition=0
      settings: InputPortMap=u0,p1
  Set J : Outport
  Set J1 : Outport  Port=2
  Set J2 : Outport  Port=3
  Set J3 : Outport  Port=4
  Out5 : Outport  Port=5
  Out6 : Outport  Port=6
  Out7 : Outport  Port=7
  Out8 : Outport  Port=8
  wires:
  Delay57/1 -> Set J/1, Delay1/1
  Delay1/1 -> Delay4/1, Set J1/1
  Delay4/1 -> Delay5/1, Set J2/1
  Delay5/1 -> Delay2/1, Set J3/1
  Delay2/1 -> Delay3/1, Out5/1
  Delay3/1 -> Delay6/1, Out6/1
  Delay6/1 -> Delay7/1, Out7/1
  Delay7/1 -> Out8/1
  data/1 -> Delay57/1
  delay/1 -> Delay7/2, Delay6/2, Delay3/2, Delay2/2, Delay5/2, Delay4/2, Delay1/2, Delay57/2

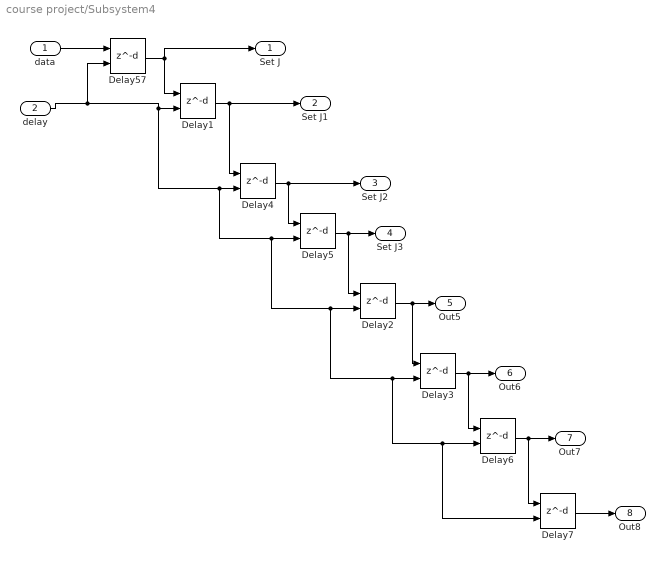
== system course project/Subsystem4 ==
  data : Inport
  delay : Inport  Port=2
  Delay{1..7,57} (8 alike) : Delay  DelayLengthSource=Input port  DelayLength=1  DelayLengthUpperLimit=2000  InitialCondition=0
      settings: InputPortMap=u0,p1
  Set J : Outport
  Set J1 : Outport  Port=2
  Set J2 : Outport  Port=3
  Set J3 : Outport  Port=4
  Out5 : Outport  Port=5
  Out6 : Outport  Port=6
  Out7 : Outport  Port=7
  Out8 : Outport  Port=8
  wires:
  Delay57/1 -> Set J/1, Delay1/1
  Delay1/1 -> Delay4/1, Set J1/1
  Delay4/1 -> Delay5/1, Set J2/1
  Delay5/1 -> Delay2/1, Set J3/1
  Delay2/1 -> Delay3/1, Out5/1
  Delay3/1 -> Delay6/1, Out6/1
  Delay6/1 -> Delay7/1, Out7/1
  Delay7/1 -> Out8/1
  data/1 -> Delay57/1
  delay/1 -> Delay7/2, Delay6/2, Delay3/2, Delay2/2, Delay5/2, Delay4/2, Delay1/2, Delay57/2

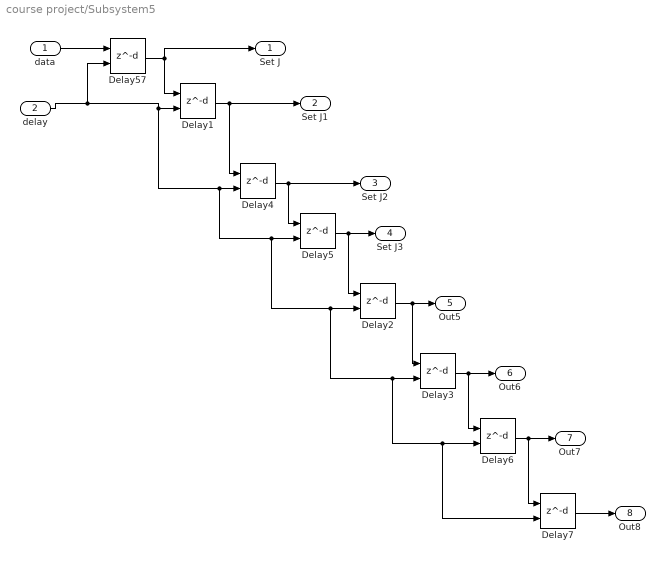
== system course project/Subsystem5 ==
  data : Inport
  delay : Inport  Port=2
  Delay{1..7,57} (8 alike) : Delay  DelayLengthSource=Input port  DelayLength=1  DelayLengthUpperLimit=2000  InitialCondition=0
      settings: InputPortMap=u0,p1
  Set J : Outport
  Set J1 : Outport  Port=2
  Set J2 : Outport  Port=3
  Set J3 : Outport  Port=4
  Out5 : Outport  Port=5
  Out6 : Outport  Port=6
  Out7 : Outport  Port=7
  Out8 : Outport  Port=8
  wires:
  Delay57/1 -> Set J/1, Delay1/1
  Delay1/1 -> Delay4/1, Set J1/1
  Delay4/1 -> Delay5/1, Set J2/1
  Delay5/1 -> Delay2/1, Set J3/1
  Delay2/1 -> Delay3/1, Out5/1
  Delay3/1 -> Delay6/1, Out6/1
  Delay6/1 -> Delay7/1, Out7/1
  Delay7/1 -> Out8/1
  data/1 -> Delay57/1
  delay/1 -> Delay7/2, Delay6/2, Delay3/2, Delay2/2, Delay5/2, Delay4/2, Delay1/2, Delay57/2

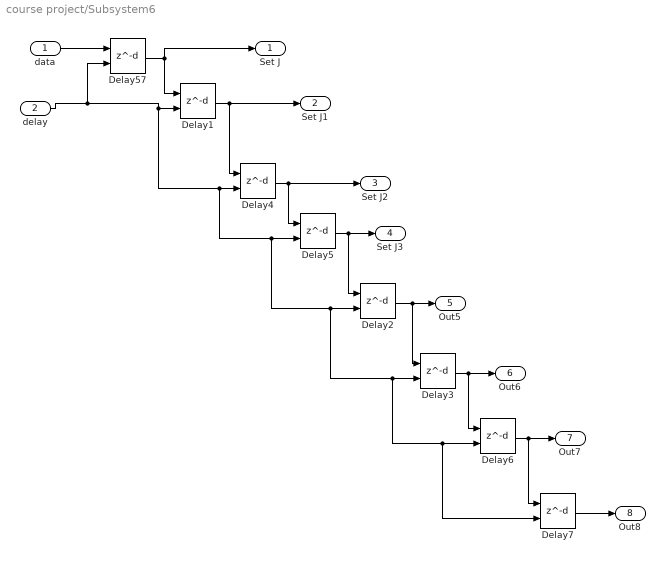
== system course project/Subsystem6 ==
  data : Inport
  delay : Inport  Port=2
  Delay{1..7,57} (8 alike) : Delay  DelayLengthSource=Input port  DelayLength=1  DelayLengthUpperLimit=2000  InitialCondition=0
      settings: InputPortMap=u0,p1
  Set J : Outport
  Set J1 : Outport  Port=2
  Set J2 : Outport  Port=3
  Set J3 : Outport  Port=4
  Out5 : Outport  Port=5
  Out6 : Outport  Port=6
  Out7 : Outport  Port=7
  Out8 : Outport  Port=8
  wires:
  Delay57/1 -> Set J/1, Delay1/1
  Delay1/1 -> Delay4/1, Set J1/1
  Delay4/1 -> Delay5/1, Set J2/1
  Delay5/1 -> Delay2/1, Set J3/1
  Delay2/1 -> Delay3/1, Out5/1
  Delay3/1 -> Delay6/1, Out6/1
  Delay6/1 -> Delay7/1, Out7/1
  Delay7/1 -> Out8/1
  data/1 -> Delay57/1
  delay/1 -> Delay7/2, Delay6/2, Delay3/2, Delay2/2, Delay5/2, Delay4/2, Delay1/2, Delay57/2

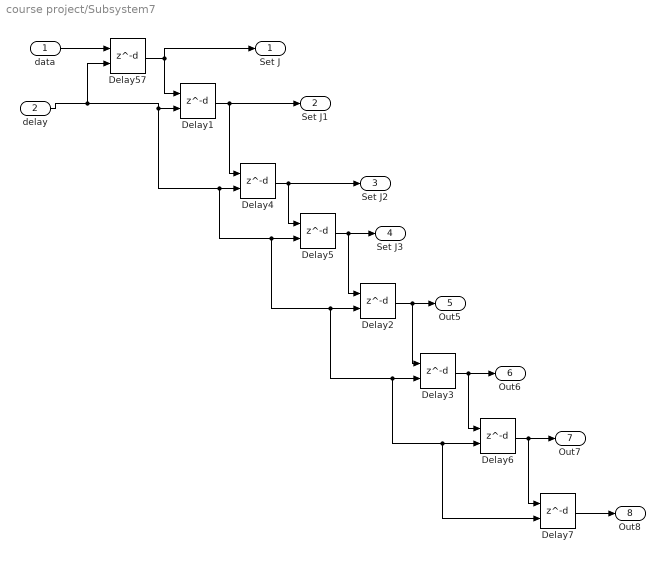
== system course project/Subsystem7 ==
  data : Inport
  delay : Inport  Port=2
  Delay{1..7,57} (8 alike) : Delay  DelayLengthSource=Input port  DelayLength=1  DelayLengthUpperLimit=2000  InitialCondition=0
      settings: InputPortMap=u0,p1
  Set J : Outport
  Set J1 : Outport  Port=2
  Set J2 : Outport  Port=3
  Set J3 : Outport  Port=4
  Out5 : Outport  Port=5
  Out6 : Outport  Port=6
  Out7 : Outport  Port=7
  Out8 : Outport  Port=8
  wires:
  Delay57/1 -> Set J/1, Delay1/1
  Delay1/1 -> Delay4/1, Set J1/1
  Delay4/1 -> Delay5/1, Set J2/1
  Delay5/1 -> Delay2/1, Set J3/1
  Delay2/1 -> Delay3/1, Out5/1
  Delay3/1 -> Delay6/1, Out6/1
  Delay6/1 -> Delay7/1, Out7/1
  Delay7/1 -> Out8/1
  data/1 -> Delay57/1
  delay/1 -> Delay7/2, Delay6/2, Delay3/2, Delay2/2, Delay5/2, Delay4/2, Delay1/2, Delay57/2

== system course project/Register/JCK-Trigger ==
  Set J : Inport
  Control C : Inport  Port=2
  Reset K : Inport  Port=3
  Logical Operator1 : Logic  Operator=NAND  Inputs=3  AllPortsSameDT=off  OutDataTypeStr=boolean
  Logical Operator2 : Logic  Operator=NAND  AllPortsSameDT=off  OutDataTypeStr=boolean
  Logical Operator3 : Logic  Operator=NAND  AllPortsSameDT=off  OutDataTypeStr=boolean
  Logical Operator5 : Logic  Operator=NAND  Inputs=3  AllPortsSameDT=off  OutDataTypeStr=boolean
  Memory : Memory
  Non-Inverted : Outport
  wires:
  Memory/1 -> Logical Operator5/2, Logical Operator3/1  "Feedback"
  Logical Operator1/1 -> Logical Operator2/1  "R"
  Logical Operator2/1 -> Non-Inverted/1, Memory/1
  Logical Operator3/1 -> Logical Operator1/2, Logical Operator2/2  "Feedback"
  Logical Operator5/1 -> Logical Operator3/2
  Set J/1 -> Logical Operator1/1
  Reset K/1 -> Logical Operator5/1
  Control C/1 -> Logical Operator5/3, Logical Operator1/3

== system course project/Register/JCK-Trigger1 ==
  Set J : Inport
  Control C : Inport  Port=2
  Reset K : Inport  Port=3
  Logical Operator1 : Logic  Operator=NAND  Inputs=3  AllPortsSameDT=off  OutDataTypeStr=boolean
  Logical Operator2 : Logic  Operator=NAND  AllPortsSameDT=off  OutDataTypeStr=boolean
  Logical Operator3 : Logic  Operator=NAND  AllPortsSameDT=off  OutDataTypeStr=boolean
  Logical Operator5 : Logic  Operator=NAND  Inputs=3  AllPortsSameDT=off  OutDataTypeStr=boolean
  Memory : Memory
  Non-Inverted : Outport
  wires:
  Memory/1 -> Logical Operator5/2, Logical Operator3/1  "Feedback"
  Logical Operator1/1 -> Logical Operator2/1  "R"
  Logical Operator2/1 -> Non-Inverted/1, Memory/1
  Logical Operator3/1 -> Logical Operator1/2, Logical Operator2/2  "Feedback"
  Logical Operator5/1 -> Logical Operator3/2
  Set J/1 -> Logical Operator1/1
  Reset K/1 -> Logical Operator5/1
  Control C/1 -> Logical Operator5/3, Logical Operator1/3

== system course project/Register/JCK-Trigger2 ==
  Set J : Inport
  Control C : Inport  Port=2
  Reset K : Inport  Port=3
  Logical Operator1 : Logic  Operator=NAND  Inputs=3  AllPortsSameDT=off  OutDataTypeStr=boolean
  Logical Operator2 : Logic  Operator=NAND  AllPortsSameDT=off  OutDataTypeStr=boolean
  Logical Operator3 : Logic  Operator=NAND  AllPortsSameDT=off  OutDataTypeStr=boolean
  Logical Operator5 : Logic  Operator=NAND  Inputs=3  AllPortsSameDT=off  OutDataTypeStr=boolean
  Memory : Memory
  Non-Inverted : Outport
  wires:
  Memory/1 -> Logical Operator5/2, Logical Operator3/1  "Feedback"
  Logical Operator1/1 -> Logical Operator2/1  "R"
  Logical Operator2/1 -> Non-Inverted/1, Memory/1
  Logical Operator3/1 -> Logical Operator1/2, Logical Operator2/2  "Feedback"
  Logical Operator5/1 -> Logical Operator3/2
  Set J/1 -> Logical Operator1/1
  Reset K/1 -> Logical Operator5/1
  Control C/1 -> Logical Operator5/3, Logical Operator1/3

== system course project/Register/JCK-Trigger3 ==
  Set J : Inport
  Control C : Inport  Port=2
  Reset K : Inport  Port=3
  Logical Operator1 : Logic  Operator=NAND  Inputs=3  AllPortsSameDT=off  OutDataTypeStr=boolean
  Logical Operator2 : Logic  Operator=NAND  AllPortsSameDT=off  OutDataTypeStr=boolean
  Logical Operator3 : Logic  Operator=NAND  AllPortsSameDT=off  OutDataTypeStr=boolean
  Logical Operator5 : Logic  Operator=NAND  Inputs=3  AllPortsSameDT=off  OutDataTypeStr=boolean
  Memory : Memory
  Non-Inverted : Outport
  wires:
  Memory/1 -> Logical Operator5/2, Logical Operator3/1  "Feedback"
  Logical Operator1/1 -> Logical Operator2/1  "R"
  Logical Operator2/1 -> Non-Inverted/1, Memory/1
  Logical Operator3/1 -> Logical Operator1/2, Logical Operator2/2  "Feedback"
  Logical Operator5/1 -> Logical Operator3/2
  Set J/1 -> Logical Operator1/1
  Reset K/1 -> Logical Operator5/1
  Control C/1 -> Logical Operator5/3, Logical Operator1/3

== system course project/Register1/JCK-Trigger ==
  Set J : Inport
  Control C : Inport  Port=2
  Reset K : Inport  Port=3
  Logical Operator1 : Logic  Operator=NAND  Inputs=3  AllPortsSameDT=off  OutDataTypeStr=boolean
  Logical Operator2 : Logic  Operator=NAND  AllPortsSameDT=off  OutDataTypeStr=boolean
  Logical Operator3 : Logic  Operator=NAND  AllPortsSameDT=off  OutDataTypeStr=boolean
  Logical Operator5 : Logic  Operator=NAND  Inputs=3  AllPortsSameDT=off  OutDataTypeStr=boolean
  Memory : Memory
  Non-Inverted : Outport
  wires:
  Memory/1 -> Logical Operator5/2, Logical Operator3/1  "Feedback"
  Logical Operator1/1 -> Logical Operator2/1  "R"
  Logical Operator2/1 -> Non-Inverted/1, Memory/1
  Logical Operator3/1 -> Logical Operator1/2, Logical Operator2/2  "Feedback"
  Logical Operator5/1 -> Logical Operator3/2
  Set J/1 -> Logical Operator1/1
  Reset K/1 -> Logical Operator5/1
  Control C/1 -> Logical Operator5/3, Logical Operator1/3

== system course project/Register1/JCK-Trigger1 ==
  Set J : Inport
  Control C : Inport  Port=2
  Reset K : Inport  Port=3
  Logical Operator1 : Logic  Operator=NAND  Inputs=3  AllPortsSameDT=off  OutDataTypeStr=boolean
  Logical Operator2 : Logic  Operator=NAND  AllPortsSameDT=off  OutDataTypeStr=boolean
  Logical Operator3 : Logic  Operator=NAND  AllPortsSameDT=off  OutDataTypeStr=boolean
  Logical Operator5 : Logic  Operator=NAND  Inputs=3  AllPortsSameDT=off  OutDataTypeStr=boolean
  Memory : Memory
  Non-Inverted : Outport
  wires:
  Memory/1 -> Logical Operator5/2, Logical Operator3/1  "Feedback"
  Logical Operator1/1 -> Logical Operator2/1  "R"
  Logical Operator2/1 -> Non-Inverted/1, Memory/1
  Logical Operator3/1 -> Logical Operator1/2, Logical Operator2/2  "Feedback"
  Logical Operator5/1 -> Logical Operator3/2
  Set J/1 -> Logical Operator1/1
  Reset K/1 -> Logical Operator5/1
  Control C/1 -> Logical Operator5/3, Logical Operator1/3

== system course project/Register1/JCK-Trigger2 ==
  Set J : Inport
  Control C : Inport  Port=2
  Reset K : Inport  Port=3
  Logical Operator1 : Logic  Operator=NAND  Inputs=3  AllPortsSameDT=off  OutDataTypeStr=boolean
  Logical Operator2 : Logic  Operator=NAND  AllPortsSameDT=off  OutDataTypeStr=boolean
  Logical Operator3 : Logic  Operator=NAND  AllPortsSameDT=off  OutDataTypeStr=boolean
  Logical Operator5 : Logic  Operator=NAND  Inputs=3  AllPortsSameDT=off  OutDataTypeStr=boolean
  Memory : Memory
  Non-Inverted : Outport
  wires:
  Memory/1 -> Logical Operator5/2, Logical Operator3/1  "Feedback"
  Logical Operator1/1 -> Logical Operator2/1  "R"
  Logical Operator2/1 -> Non-Inverted/1, Memory/1
  Logical Operator3/1 -> Logical Operator1/2, Logical Operator2/2  "Feedback"
  Logical Operator5/1 -> Logical Operator3/2
  Set J/1 -> Logical Operator1/1
  Reset K/1 -> Logical Operator5/1
  Control C/1 -> Logical Operator5/3, Logical Operator1/3

== system course project/Register1/JCK-Trigger3 ==
  Set J : Inport
  Control C : Inport  Port=2
  Reset K : Inport  Port=3
  Logical Operator1 : Logic  Operator=NAND  Inputs=3  AllPortsSameDT=off  OutDataTypeStr=boolean
  Logical Operator2 : Logic  Operator=NAND  AllPortsSameDT=off  OutDataTypeStr=boolean
  Logical Operator3 : Logic  Operator=NAND  AllPortsSameDT=off  OutDataTypeStr=boolean
  Logical Operator5 : Logic  Operator=NAND  Inputs=3  AllPortsSameDT=off  OutDataTypeStr=boolean
  Memory : Memory
  Non-Inverted : Outport
  wires:
  Memory/1 -> Logical Operator5/2, Logical Operator3/1  "Feedback"
  Logical Operator1/1 -> Logical Operator2/1  "R"
  Logical Operator2/1 -> Non-Inverted/1, Memory/1
  Logical Operator3/1 -> Logical Operator1/2, Logical Operator2/2  "Feedback"
  Logical Operator5/1 -> Logical Operator3/2
  Set J/1 -> Logical Operator1/1
  Reset K/1 -> Logical Operator5/1
  Control C/1 -> Logical Operator5/3, Logical Operator1/3

== system course project/Register10/JCK-Trigger ==
  Set J : Inport
  Control C : Inport  Port=2
  Reset K : Inport  Port=3
  Logical Operator1 : Logic  Operator=NAND  Inputs=3  AllPortsSameDT=off  OutDataTypeStr=boolean
  Logical Operator2 : Logic  Operator=NAND  AllPortsSameDT=off  OutDataTypeStr=boolean
  Logical Operator3 : Logic  Operator=NAND  AllPortsSameDT=off  OutDataTypeStr=boolean
  Logical Operator5 : Logic  Operator=NAND  Inputs=3  AllPortsSameDT=off  OutDataTypeStr=boolean
  Memory : Memory
  Non-Inverted : Outport
  wires:
  Memory/1 -> Logical Operator5/2, Logical Operator3/1  "Feedback"
  Logical Operator1/1 -> Logical Operator2/1  "R"
  Logical Operator2/1 -> Non-Inverted/1, Memory/1
  Logical Operator3/1 -> Logical Operator1/2, Logical Operator2/2  "Feedback"
  Logical Operator5/1 -> Logical Operator3/2
  Set J/1 -> Logical Operator1/1
  Reset K/1 -> Logical Operator5/1
  Control C/1 -> Logical Operator5/3, Logical Operator1/3

== system course project/Register10/JCK-Trigger1 ==
  Set J : Inport
  Control C : Inport  Port=2
  Reset K : Inport  Port=3
  Logical Operator1 : Logic  Operator=NAND  Inputs=3  AllPortsSameDT=off  OutDataTypeStr=boolean
  Logical Operator2 : Logic  Operator=NAND  AllPortsSameDT=off  OutDataTypeStr=boolean
  Logical Operator3 : Logic  Operator=NAND  AllPortsSameDT=off  OutDataTypeStr=boolean
  Logical Operator5 : Logic  Operator=NAND  Inputs=3  AllPortsSameDT=off  OutDataTypeStr=boolean
  Memory : Memory
  Non-Inverted : Outport
  wires:
  Memory/1 -> Logical Operator5/2, Logical Operator3/1  "Feedback"
  Logical Operator1/1 -> Logical Operator2/1  "R"
  Logical Operator2/1 -> Non-Inverted/1, Memory/1
  Logical Operator3/1 -> Logical Operator1/2, Logical Operator2/2  "Feedback"
  Logical Operator5/1 -> Logical Operator3/2
  Set J/1 -> Logical Operator1/1
  Reset K/1 -> Logical Operator5/1
  Control C/1 -> Logical Operator5/3, Logical Operator1/3

== system course project/Register10/JCK-Trigger2 ==
  Set J : Inport
  Control C : Inport  Port=2
  Reset K : Inport  Port=3
  Logical Operator1 : Logic  Operator=NAND  Inputs=3  AllPortsSameDT=off  OutDataTypeStr=boolean
  Logical Operator2 : Logic  Operator=NAND  AllPortsSameDT=off  OutDataTypeStr=boolean
  Logical Operator3 : Logic  Operator=NAND  AllPortsSameDT=off  OutDataTypeStr=boolean
  Logical Operator5 : Logic  Operator=NAND  Inputs=3  AllPortsSameDT=off  OutDataTypeStr=boolean
  Memory : Memory
  Non-Inverted : Outport
  wires:
  Memory/1 -> Logical Operator5/2, Logical Operator3/1  "Feedback"
  Logical Operator1/1 -> Logical Operator2/1  "R"
  Logical Operator2/1 -> Non-Inverted/1, Memory/1
  Logical Operator3/1 -> Logical Operator1/2, Logical Operator2/2  "Feedback"
  Logical Operator5/1 -> Logical Operator3/2
  Set J/1 -> Logical Operator1/1
  Reset K/1 -> Logical Operator5/1
  Control C/1 -> Logical Operator5/3, Logical Operator1/3

== system course project/Register10/JCK-Trigger3 ==
  Set J : Inport
  Control C : Inport  Port=2
  Reset K : Inport  Port=3
  Logical Operator1 : Logic  Operator=NAND  Inputs=3  AllPortsSameDT=off  OutDataTypeStr=boolean
  Logical Operator2 : Logic  Operator=NAND  AllPortsSameDT=off  OutDataTypeStr=boolean
  Logical Operator3 : Logic  Operator=NAND  AllPortsSameDT=off  OutDataTypeStr=boolean
  Logical Operator5 : Logic  Operator=NAND  Inputs=3  AllPortsSameDT=off  OutDataTypeStr=boolean
  Memory : Memory
  Non-Inverted : Outport
  wires:
  Memory/1 -> Logical Operator5/2, Logical Operator3/1  "Feedback"
  Logical Operator1/1 -> Logical Operator2/1  "R"
  Logical Operator2/1 -> Non-Inverted/1, Memory/1
  Logical Operator3/1 -> Logical Operator1/2, Logical Operator2/2  "Feedback"
  Logical Operator5/1 -> Logical Operator3/2
  Set J/1 -> Logical Operator1/1
  Reset K/1 -> Logical Operator5/1
  Control C/1 -> Logical Operator5/3, Logical Operator1/3

== system course project/Register11/JCK-Trigger ==
  Set J : Inport
  Control C : Inport  Port=2
  Reset K : Inport  Port=3
  Logical Operator1 : Logic  Operator=NAND  Inputs=3  AllPortsSameDT=off  OutDataTypeStr=boolean
  Logical Operator2 : Logic  Operator=NAND  AllPortsSameDT=off  OutDataTypeStr=boolean
  Logical Operator3 : Logic  Operator=NAND  AllPortsSameDT=off  OutDataTypeStr=boolean
  Logical Operator5 : Logic  Operator=NAND  Inputs=3  AllPortsSameDT=off  OutDataTypeStr=boolean
  Memory : Memory
  Non-Inverted : Outport
  wires:
  Memory/1 -> Logical Operator5/2, Logical Operator3/1  "Feedback"
  Logical Operator1/1 -> Logical Operator2/1  "R"
  Logical Operator2/1 -> Non-Inverted/1, Memory/1
  Logical Operator3/1 -> Logical Operator1/2, Logical Operator2/2  "Feedback"
  Logical Operator5/1 -> Logical Operator3/2
  Set J/1 -> Logical Operator1/1
  Reset K/1 -> Logical Operator5/1
  Control C/1 -> Logical Operator5/3, Logical Operator1/3

== system course project/Register11/JCK-Trigger1 ==
  Set J : Inport
  Control C : Inport  Port=2
  Reset K : Inport  Port=3
  Logical Operator1 : Logic  Operator=NAND  Inputs=3  AllPortsSameDT=off  OutDataTypeStr=boolean
  Logical Operator2 : Logic  Operator=NAND  AllPortsSameDT=off  OutDataTypeStr=boolean
  Logical Operator3 : Logic  Operator=NAND  AllPortsSameDT=off  OutDataTypeStr=boolean
  Logical Operator5 : Logic  Operator=NAND  Inputs=3  AllPortsSameDT=off  OutDataTypeStr=boolean
  Memory : Memory
  Non-Inverted : Outport
  wires:
  Memory/1 -> Logical Operator5/2, Logical Operator3/1  "Feedback"
  Logical Operator1/1 -> Logical Operator2/1  "R"
  Logical Operator2/1 -> Non-Inverted/1, Memory/1
  Logical Operator3/1 -> Logical Operator1/2, Logical Operator2/2  "Feedback"
  Logical Operator5/1 -> Logical Operator3/2
  Set J/1 -> Logical Operator1/1
  Reset K/1 -> Logical Operator5/1
  Control C/1 -> Logical Operator5/3, Logical Operator1/3

== system course project/Register11/JCK-Trigger2 ==
  Set J : Inport
  Control C : Inport  Port=2
  Reset K : Inport  Port=3
  Logical Operator1 : Logic  Operator=NAND  Inputs=3  AllPortsSameDT=off  OutDataTypeStr=boolean
  Logical Operator2 : Logic  Operator=NAND  AllPortsSameDT=off  OutDataTypeStr=boolean
  Logical Operator3 : Logic  Operator=NAND  AllPortsSameDT=off  OutDataTypeStr=boolean
  Logical Operator5 : Logic  Operator=NAND  Inputs=3  AllPortsSameDT=off  OutDataTypeStr=boolean
  Memory : Memory
  Non-Inverted : Outport
  wires:
  Memory/1 -> Logical Operator5/2, Logical Operator3/1  "Feedback"
  Logical Operator1/1 -> Logical Operator2/1  "R"
  Logical Operator2/1 -> Non-Inverted/1, Memory/1
  Logical Operator3/1 -> Logical Operator1/2, Logical Operator2/2  "Feedback"
  Logical Operator5/1 -> Logical Operator3/2
  Set J/1 -> Logical Operator1/1
  Reset K/1 -> Logical Operator5/1
  Control C/1 -> Logical Operator5/3, Logical Operator1/3

== system course project/Register11/JCK-Trigger3 ==
  Set J : Inport
  Control C : Inport  Port=2
  Reset K : Inport  Port=3
  Logical Operator1 : Logic  Operator=NAND  Inputs=3  AllPortsSameDT=off  OutDataTypeStr=boolean
  Logical Operator2 : Logic  Operator=NAND  AllPortsSameDT=off  OutDataTypeStr=boolean
  Logical Operator3 : Logic  Operator=NAND  AllPortsSameDT=off  OutDataTypeStr=boolean
  Logical Operator5 : Logic  Operator=NAND  Inputs=3  AllPortsSameDT=off  OutDataTypeStr=boolean
  Memory : Memory
  Non-Inverted : Outport
  wires:
  Memory/1 -> Logical Operator5/2, Logical Operator3/1  "Feedback"
  Logical Operator1/1 -> Logical Operator2/1  "R"
  Logical Operator2/1 -> Non-Inverted/1, Memory/1
  Logical Operator3/1 -> Logical Operator1/2, Logical Operator2/2  "Feedback"
  Logical Operator5/1 -> Logical Operator3/2
  Set J/1 -> Logical Operator1/1
  Reset K/1 -> Logical Operator5/1
  Control C/1 -> Logical Operator5/3, Logical Operator1/3

== system course project/Register12/JCK-Trigger ==
  Set J : Inport
  Control C : Inport  Port=2
  Reset K : Inport  Port=3
  Logical Operator1 : Logic  Operator=NAND  Inputs=3  AllPortsSameDT=off  OutDataTypeStr=boolean
  Logical Operator2 : Logic  Operator=NAND  AllPortsSameDT=off  OutDataTypeStr=boolean
  Logical Operator3 : Logic  Operator=NAND  AllPortsSameDT=off  OutDataTypeStr=boolean
  Logical Operator5 : Logic  Operator=NAND  Inputs=3  AllPortsSameDT=off  OutDataTypeStr=boolean
  Memory : Memory
  Non-Inverted : Outport
  wires:
  Memory/1 -> Logical Operator5/2, Logical Operator3/1  "Feedback"
  Logical Operator1/1 -> Logical Operator2/1  "R"
  Logical Operator2/1 -> Non-Inverted/1, Memory/1
  Logical Operator3/1 -> Logical Operator1/2, Logical Operator2/2  "Feedback"
  Logical Operator5/1 -> Logical Operator3/2
  Set J/1 -> Logical Operator1/1
  Reset K/1 -> Logical Operator5/1
  Control C/1 -> Logical Operator5/3, Logical Operator1/3

== system course project/Register12/JCK-Trigger1 ==
  Set J : Inport
  Control C : Inport  Port=2
  Reset K : Inport  Port=3
  Logical Operator1 : Logic  Operator=NAND  Inputs=3  AllPortsSameDT=off  OutDataTypeStr=boolean
  Logical Operator2 : Logic  Operator=NAND  AllPortsSameDT=off  OutDataTypeStr=boolean
  Logical Operator3 : Logic  Operator=NAND  AllPortsSameDT=off  OutDataTypeStr=boolean
  Logical Operator5 : Logic  Operator=NAND  Inputs=3  AllPortsSameDT=off  OutDataTypeStr=boolean
  Memory : Memory
  Non-Inverted : Outport
  wires:
  Memory/1 -> Logical Operator5/2, Logical Operator3/1  "Feedback"
  Logical Operator1/1 -> Logical Operator2/1  "R"
  Logical Operator2/1 -> Non-Inverted/1, Memory/1
  Logical Operator3/1 -> Logical Operator1/2, Logical Operator2/2  "Feedback"
  Logical Operator5/1 -> Logical Operator3/2
  Set J/1 -> Logical Operator1/1
  Reset K/1 -> Logical Operator5/1
  Control C/1 -> Logical Operator5/3, Logical Operator1/3
